simulink model "simulateBPSK_pulseShapingRectangular_variableNoise"  (R2017a)
settings: Solver=VariableStepAuto  StartTime=0.0  StopTime=inf  RelTol=1e-3
InitFcn:
  | Tb = 0.001;
  | fs = 1e4;
  | Ts = 1/fs;
  | frameSize = 1000;
libraries: commdigbbndpm3 x2, commfilt2 x2, commchan3 x1, commrandsrc3 x1, commsink2 x1, simulink x1
settings Model: Creator=prust  LastModifiedBy=prust

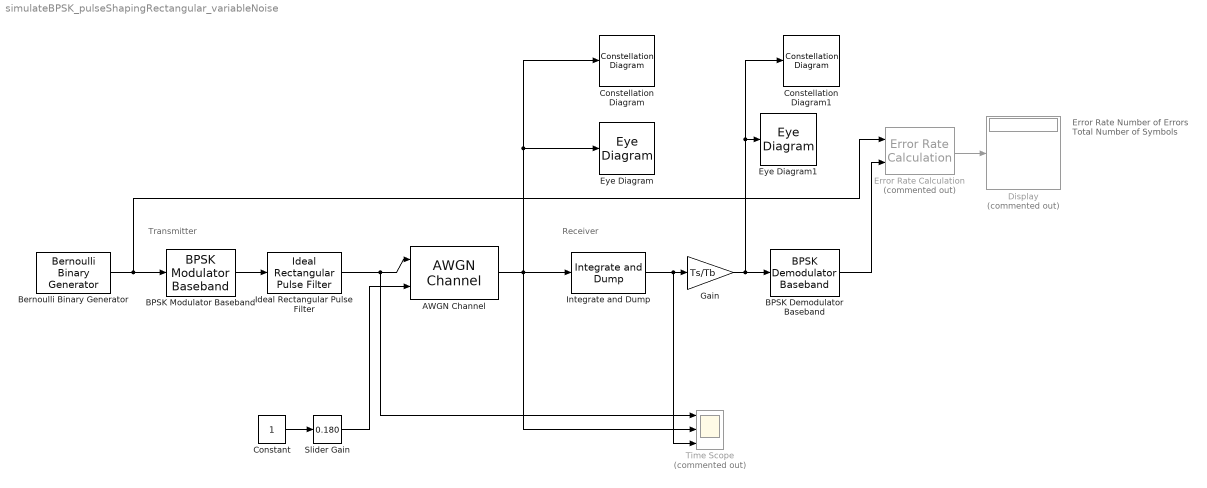
== system simulateBPSK_pulseShapingRectangular_variableNoise ==
  note: Receiver
  note: Transmitter
  note: Error Rate
      |
      | Number of Errors
      |
      | Total Number of Symbols
  AWGN Channel : commchan3/AWGN Channel  InputProcessing=Columns as channels (frame based)  seed=67  noiseMode=Variance from port  EbNodB=16  EsNodB=10  SNRdB=10  bitsPerSym=1  Ps=1  Tsym=Tb  variance=1
  BPSK Demodulator Baseband : commdigbbndpm3/BPSK Demodulator Baseband  DecType=Hard decision  VarSource=Dialog  Variance=1  Ph=0  outDtype=Inherit via internal rule  derotateFactorWordLen=16  derotateFactorDataTypeStr=Inherit: Same word length as input  derotateFactorLastDataTypeStr=Inherit: Same word length as input
  BPSK Modulator Baseband : commdigbbndpm3/BPSK Modulator Baseband  Ph=0  outDtype=double  outWordLen=16  outUDDataType=sfix(16)  outFracLenMode=Best precision  outFracLen=15  outDataTypeStr=double  outLastDataTypeStr=double
  Bernoulli Binary Generator : commrandsrc3/Bernoulli Binary Generator  ProbabilityOfZero=0.5  SeedSource=Auto  Seed=0  SampleTime=Tb  SamplesPerFrame=frameSize  OutputDataType=double  SimulateUsing=Interpreted execution
  Constant : Constant
  Constellation Diagram : ConstellationDiagram
  Constellation Diagram1 : ConstellationDiagram
  Display : Display  Commented=on
  Error Rate Calculation : commsink2/Error Rate Calculation  Commented=on  N=0  st_delay=0  cp_mode=Entire frame  subframe=[]  PMode=Port  WsName=ErrorVec  RsMode2=off  stop=off  numErr=100  maxBits=1e6
  Eye Diagram : EyeDiagram
  Eye Diagram1 : EyeDiagram
  Gain : Gain  Gain=Ts/Tb
  Ideal Rectangular Pulse Filter : commfilt2/Ideal Rectangular Pulse Filter  pulseLen=Tb/Ts  pulseDelay=0  InputProcessing=Columns as channels (frame based)  RateOptions=Enforce single-rate processing  sampMode=Mute  normCheck=off  normMode=Sum of samples  filterGain=1  saveAsFlag=0  roundingMode=Floor  overflowMode=off  firstCoeffDataTypeStr=Inherit: Same word length as input  firstCoeffMin=[]  firstCoeffMax=[]  firstCoeffLastDataTypeStr=Inherit: Same word length as input  outputDataTypeStr=Inherit: Same as accumulator  outputMin=[]  outputMax=[]  outputLastDataTypeStr=Inherit: Same as accumulator
      settings: SourceProductName=Communications System Toolbox  SourceProductBaseCode=CM
  Integrate and Dump : commfilt2/Integrate and Dump  obssamples=Tb/Ts  offsetsamples=0  nodump=off  roundingMode=Floor  overflowMode=off  outputDataTypeStr=Inherit: Same as accumulator  outputLastDataTypeStr=Inherit: Same as accumulator
      settings: SourceProductName=Communications System Toolbox
  Slider Gain : simulink/Math Operations/Slider Gain  gain=0.180  low=0  high=2
  Time Scope : Scope  Commented=on  NumInputPorts=3
  wires:
  Bernoulli Binary Generator/1 -> Error Rate Calculation/1, BPSK Modulator Baseband/1
  AWGN Channel/1 -> Integrate and Dump/1, Constellation Diagram/1, Eye Diagram/1, Time Scope/2
  BPSK Demodulator Baseband/1 -> Error Rate Calculation/2
  Error Rate Calculation/1 -> Display/1
  Ideal Rectangular Pulse Filter/1 -> AWGN Channel/1, Time Scope/1
  Integrate and Dump/1 -> Time Scope/3, Gain/1
  BPSK Modulator Baseband/1 -> Ideal Rectangular Pulse Filter/1
  Gain/1 -> Eye Diagram1/1, Constellation Diagram1/1, BPSK Demodulator Baseband/1
  Constant/1 -> Slider Gain/1
  Slider Gain/1 -> AWGN Channel/2
